simulink model "simulink"  (R2015a)
settings: Solver=ode4  StartTime=0.0  StopTime=inf  FixedStep=1e-3  RelTol=1e-3
values from neighbouring files (symbols this model uses):
  b_end1 = 0.5*(k_end1*Cyl1.m)^0.5    [m-script.m]
  b_end2 = 0.5*(k_end2*Cyl2.m)^0.5    [m-script.m]
  b_end3 = 0.5*(k_end3*Cyl3.m)^0.5    [m-script.m]
  b_end4 = 0.5*(k_end4*Cyl4.m)^0.5    [m-script.m]
  Cyl1_b = 40000    [m-script.m]
  Cyl1_Fc = 20514    [m-script.m]
  Cyl1_Fs = 22360    [m-script.m]
  Cyl1_K = 20000    [m-script.m]
  Cyl1_vs = 0.8    [m-script.m]
  Cyl2_b = 30000    [m-script.m]
  Cyl2_Fc = 14950    [m-script.m]
  Cyl2_Fs = 16125    [m-script.m]
  Cyl2_K = 20000    [m-script.m]
  Cyl2_vs = 0.8    [m-script.m]
  Cyl3_b = 30000    [m-script.m]
  Cyl3_Fc = 14996    [m-script.m]
  Cyl3_Fs = 16340    [m-script.m]
  Cyl3_K = 20000    [m-script.m]
  Cyl3_vs = 0.8    [m-script.m]
  Cyl4_b = 8500    [m-script.m]
  Cyl4_Fc = 4570    [m-script.m]
  Cyl4_Fs = 4945    [m-script.m]
  Cyl4_K = 20000    [m-script.m]
  Cyl4_vs = 0.8    [m-script.m]
  k_end1 = (pr_Ps*Cyl1.A_A)/v1    [m-script.m]
  k_end2 = (pr_Ps*Cyl2.A_A)/v2    [m-script.m]
  k_end3 = (pr_Ps*Cyl3.A_A)/v3    [m-script.m]
  k_end4 = (pr_Ps*Cyl4.A_A)/v4    [m-script.m]
  pr_Ps = 215e5    (= 21500000)    [m-script.m]
  sampleTime = 0.001    [m-script.m]
  Valve_eta = 0.989    [m-script.m]
  Valve_omega = 40.5    [m-script.m]
undefined symbols (not defined in the file or in its folder): Cyl, Cyl1, Cyl2, Cyl3, Cyl4, Cylinder2, Cylinder3, Cylinder4, Extention1, Extention2, Lift, Link1, Pillar, Pinion, Piston2, Piston3, Piston4, Rack, Tilt, Valve, X, Y, Z
undefined symbols (not defined in the file): Valve1, Valve2, Valve3, Valve4
libraries: sm_lib x72, simulink x32, nesl_utility x20, simulink_extras x3, xpcrtudplib x2, xpcobsoletelib x2
(part 1 of 4)
settings Model: CovModelRefEnable=off  Creator=Lakshmi  LastModifiedBy=IHA2700
settings SolverCC: EnableConcurrentExecution=on
settings DataIOCC: LimitDataPoints=off  SaveFormat=Dataset
settings OptimizationCC: BlockReduction=off  OptimizeBlockIOStorage=off  BufferReuse=off  GlobalBufferReuse=off  ExpressionFolding=off  LocalBlockOutputs=off
settings HardwareCC: ProdIntDivRoundTo=Zero  ProdEndianess=LittleEndian  ProdLongLongMode=on  ProdHWDeviceType=Generic->32-bit x86 compatible
settings ModelReferenceCC: PropagateSignalLabelsOutOfModel=on
settings RTWCC: SystemTargetFile=slrt.tlc  TemplateMakefile=slrt_default_tmf  Description=Simulink Real-Time  RTWCompilerOptimization=on
settings SimulinkRealTimeCC: GeneratePreprocessorConditionals=Disable all  xPCisModelTimeout=off
settings ConfigurationSet: Description=Simscape Multibody

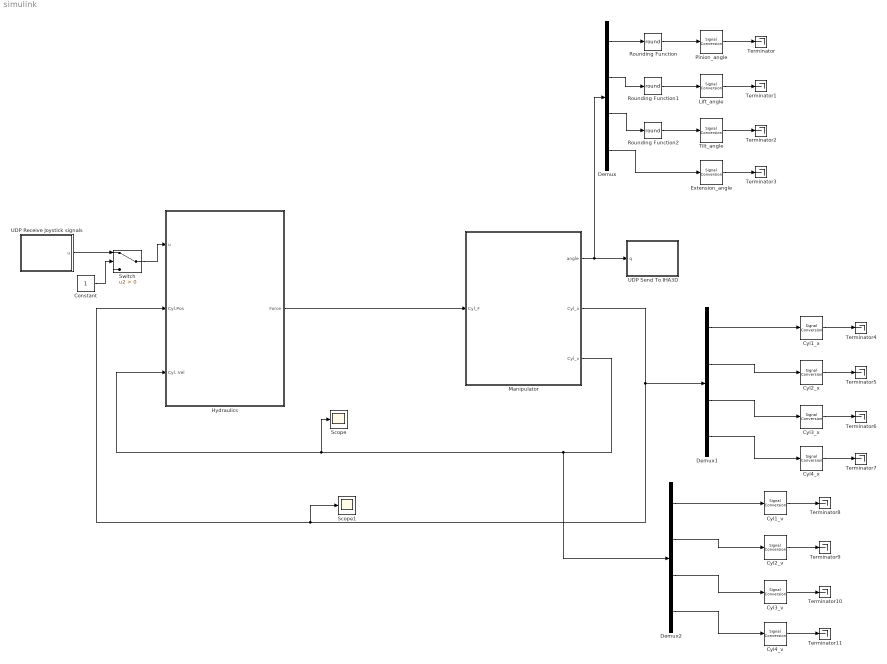
== system simulink ==
  Constant : Constant
  Cyl1_v : SignalConversion
  Cyl1_x : SignalConversion
  Cyl2_v : SignalConversion
  Cyl2_x : SignalConversion
  Cyl3_v : SignalConversion
  Cyl3_x : SignalConversion
  Cyl4_v : SignalConversion
  Cyl4_x : SignalConversion
  Demux : Demux
  Demux1 : Demux
  Demux2 : Demux
  Extension_angle : SignalConversion
  Hydraulics : Subsystem
  Lift_angle : SignalConversion
  Manipulator : Subsystem
  Pinion_angle : SignalConversion
  Rounding Function : Rounding  Operator=round
  Rounding Function1 : Rounding  Operator=round
  Rounding Function2 : Rounding  Operator=round
  Scope : Scope
      settings: YMin=-0.00025  YMax=0.00175  SaveName=ScopeData25
  Scope1 : Scope
      settings: YMin=2.77556e-17  YMax=0.7  SaveName=ScopeData26
  Switch : Switch  Criteria=u2 > Threshold
  Terminator{,1..11} (12 alike) : Terminator
  Tilt_angle : SignalConversion
  UDP Receive Joystick signals : Subsystem
  UDP Send To IHA3D : Subsystem
  wires:
  Hydraulics/1(Force) -> Manipulator/1(Cyl_F)
  Manipulator/1("angle ") -> Demux/1, UDP Send To IHA3D/1(q)
  UDP Receive Joystick signals/1(u) -> Switch/1
  Switch/1 -> Hydraulics/1(u)
  Constant/1 -> Switch/2
  Demux/1 -> Rounding Function/1
  Demux/2 -> Rounding Function1/1
  Demux/3 -> Rounding Function2/1
  Rounding Function/1 -> Pinion_angle/1
  Rounding Function1/1 -> Lift_angle/1
  Rounding Function2/1 -> Tilt_angle/1
  Demux/4 -> Extension_angle/1
  Pinion_angle/1 -> Terminator/1
  Lift_angle/1 -> Terminator1/1
  Tilt_angle/1 -> Terminator2/1
  Extension_angle/1 -> Terminator3/1
  Manipulator/2(Cyl_x) -> Demux1/1, Scope1/1, Hydraulics/2(Cyl.Pos)
  Demux1/1 -> Cyl1_x/1
  Demux1/2 -> Cyl2_x/1
  Demux1/3 -> Cyl3_x/1
  Demux1/4 -> Cyl4_x/1
  Cyl1_x/1 -> Terminator4/1
  Cyl2_x/1 -> Terminator5/1
  Cyl3_x/1 -> Terminator6/1
  Cyl4_x/1 -> Terminator7/1
  Manipulator/3(Cyl_v) -> Demux2/1, Scope/1, Hydraulics/3(Cyl. Vel)
  Demux2/1 -> Cyl1_v/1
  Demux2/2 -> Cyl2_v/1
  Demux2/3 -> Cyl3_v/1
  Demux2/4 -> Cyl4_v/1
  Cyl1_v/1 -> Terminator8/1
  Cyl2_v/1 -> Terminator9/1
  Cyl3_v/1 -> Terminator10/1
  Cyl4_v/1 -> Terminator11/1

== system simulink/Hydraulics ==
  u : Inport
  Cyl.Pos : Inport  Port=2
  Cyl. Vel : Inport  Port=3
  Constant1 : Constant  Value=pr_Ps
  Cylinder 1 : Subsystem
  Cylinder 2 : Subsystem
  Cylinder 3 : Subsystem
  Cylinder 5 : Subsystem
  Demux : Demux
  Demux1 : Demux
  Demux2 : Demux
  Mux : Mux
  Scope{,1..7} (8 alike) : Scope
      Scope settings: SaveName=ScopeData27
      Scope1 settings: YMin=0.65972  YMax=0.659805  SaveName=ScopeData28
      Scope2 settings: YMin=0.23118  YMax=0.23126  SaveName=ScopeData29
      Scope3 settings: YMin=0.359998  YMax=0.36  SaveName=ScopeData36
      Scope4 settings: SaveName=ScopeData37
      Scope5 settings: SaveName=ScopeData38
      Scope6 settings: YMin=9.845e-06  YMax=9.955e-06  SaveName=ScopeData39
      Scope7 settings: YMin=-3.8e-07  YMax=-2.5e-07  SaveName=ScopeData40
  Force : Outport
  wires:
  Cylinder 5/1(" Force") -> Mux/4
  Cyl.Pos/1 -> Demux/1
  Demux2/3 -> Scope5/1, Cylinder 3/2(v)
  Cylinder 3/1(" Force") -> Mux/3
  Cylinder 1/1(" Force") -> Mux/1
  Cylinder 2/1(" Force") -> Mux/2
  Demux/1 -> Scope3/1, Cylinder 1/3(x)
  Cyl. Vel/1 -> Demux2/1
  Demux/2 -> Scope2/1, Cylinder 2/3(x)
  Demux2/4 -> Scope4/1, Cylinder 5/2(v)
  Demux/3 -> Scope1/1, Cylinder 3/1(x)
  Mux/1 -> Force/1
  Demux2/2 -> Scope6/1, Cylinder 2/2(v)
  Demux1/1 -> Cylinder 1/1(u)
  Demux1/2 -> Cylinder 2/1(u)
  Demux1/3 -> Cylinder 3/3(u)
  Demux1/4 -> Cylinder 5/3(u)
  u/1 -> Demux1/1
  Constant1/1 -> Cylinder 2/4(Supply.Pr), Cylinder 1/4(Supply.Pr), Cylinder 5/4(Supply.Pr), Cylinder 3/4(Supply.Pr)
  Demux/4 -> Scope/1, Cylinder 5/1(x)
  Demux2/1 -> Scope7/1, Cylinder 1/2(v)

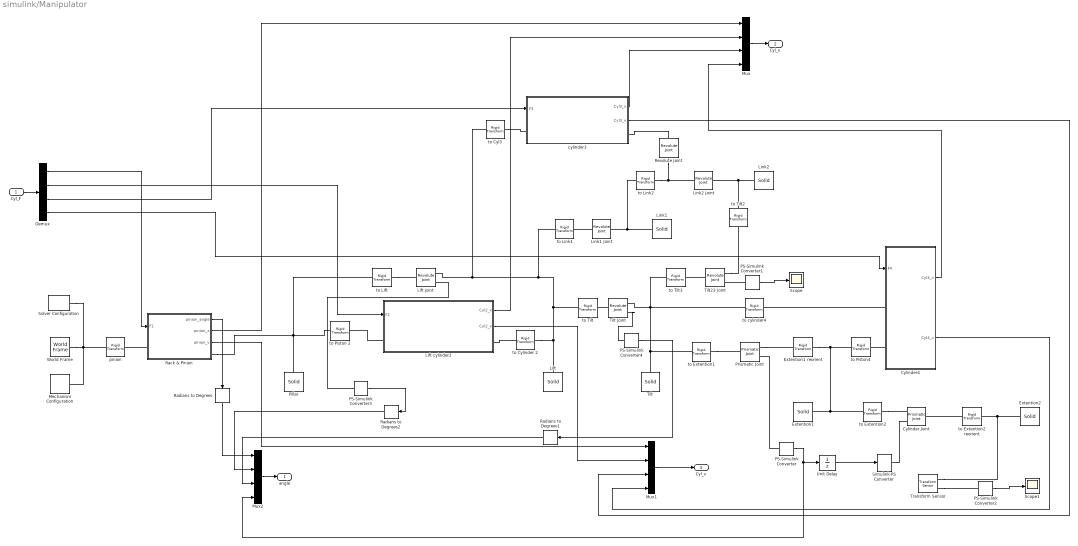
== system simulink/Manipulator ==
  Cyl_F : Inport
  Cylinder Joint : sm_lib/Joints/Prismatic Joint  SenseConstraintForce=off  SenseConstraintForceX=off  SenseConstraintForceY=off  SenseConstraintForceZ=off  SenseConstraintTorque=off  SenseConstraintTorqueX=off  SenseConstraintTorqueY=off  SenseConstraintTorqueZ=off  SenseTotalForce=off  SenseTotalForceX=off  SenseTotalForceY=off  SenseTotalForceZ=off  SenseTotalTorque=off  SenseTotalTorqueX=off  SenseTotalTorqueY=off  SenseTotalTorqueZ=off  CompositeWrenchDir=FollowerOnBase  CompositeWrenchFrame=BaseFrame  EquilibriumPosition=0  EquilibriumPositionUnits=m  SpringStiffness=0  SpringStiffnessUnits=N/m  DampingCoefficient=0  DampingCoefficientUnits=N/(m/s)  TorqueActuationMode=ComputedTorque  MotionActuationMode=InputMotion  SensePosition=off  SenseVelocity=off  SenseAcceleration=off  SenseTorqueForce=off  PositionTargetSpecify=off  PositionTargetPriority=High  PositionTargetValue=0  PositionTargetValueUnits=m  VelocityTargetSpecify=off  VelocityTargetPriority=High  VelocityTargetValue=0  VelocityTargetValueUnits=m/s  BlockFunction=simmechanics.library.joints.prismatic_joint
  Cylinder4 : Subsystem
  Demux : Demux
  Extention1 : sm_lib/Body Elements/Solid  InertiaType=Custom  Mass=Extention1.m  MassUnits=kg  CenterOfMass=Extention1.cm  CenterOfMassUnits=m  MomentsOfInertia=[1 1 1]  MomentsOfInertiaUnits=kg*m^2  ProductsOfInertia=[0 0 0]  ProductsOfInertiaUnits=kg*m^2  DensityBased=on  Density=1000  DensityUnits=kg/(m^3)  GraphicType=FromGeometry  MarkerShape=Sphere  MarkerSize=10  MarkerSizeUnits=m  GraphicVisPropType=SimpleVisualProperties  GraphicDiffuseColor=Extention1.rgb  GraphicSpecularColor=[0.5 0.5 0.5 1.0]  GraphicAmbientColor=[0.15 0.15 0.15 1.0]  GraphicEmissiveColor=[0.0 0.0 0.0 1.0]  GraphicShininess=75  GraphicOpacity=1.0  GeometryShape=GeneralExtrusion  RectangleSize=[1 1]  RectangleSizeUnits=m  BrickDimensions=[1 1 1]  BrickDimensionUnits=m  CylinderRadius=1  CylinderRadiusUnits=m  CylinderLength=1  CylinderLengthUnits=m  SphereRadius=1  SphereRadiusUnits=m  EllipsoidRadii=[1 1 1]  EllipsoidRadiiUnits=m  ExtrusionCrossSection=Extention1.c  ExtrusionCrossSectionUnits=m  ExtrusionLength=Extention1.l+0.1  ExtrusionLengthUnits=m  PolygonNumSides=3  PolygonOuterRadius=1  PolygonOuterRadiusUnits=m  ExtGeomFileType=STEP  ExtGeomFileUnits=m  RevolutionCrossSection=[1 1; 1 -1; 2 -1; 2 1]  RevolutionCrossSectionUnits=m  RevolutionExtent=Full  RevolutionAngle=180  RevolutionAngleUnits=deg  BlockFunction=simmechanics.library.body_elements.solid
  Extention1 reorient : sm_lib/Frames and Transforms/Rigid Transform  TranslationMethod=None  TranslationLengthUnit=m  TranslationStandardAxis=+Z  TranslationStandardOffset=0  TranslationCartesianOffset=Extention1.j  TranslationROffset=0  TranslationROffsetUnits=m  TranslationZOffset=0  TranslationZOffsetUnits=m  TranslationThetaOffset=0  TranslationThetaOffsetUnits=deg  RotationMethod=StandardAxis  RotationAngleUnits=deg  RotationStandardAxis=+Y  RotationAngle=-90  RotationArbitraryAxis=[0 0 1]  FollAlignAxisA=+X  BaseAlignAxisA=+Y  FollAlignAxisB=+Y  BaseAlignAxisB=+Z  RotationMatrix=[1 0 0; 0 1 0; 0 0 1]  BlockFunction=simmechanics.library.frames_transforms.rigid_transform
  Extention2 : sm_lib/Body Elements/Solid  InertiaType=Custom  Mass=Extention2.m  MassUnits=kg  CenterOfMass=Extention2.cm  CenterOfMassUnits=m  MomentsOfInertia=[1 1 1]  MomentsOfInertiaUnits=kg*m^2  ProductsOfInertia=[0 0 0]  ProductsOfInertiaUnits=kg*m^2  DensityBased=on  Density=1000  DensityUnits=kg/(m^3)  GraphicType=FromGeometry  MarkerShape=Sphere  MarkerSize=10  MarkerSizeUnits=m  GraphicVisPropType=SimpleVisualProperties  GraphicDiffuseColor=[Extention2.rgb]  GraphicSpecularColor=[0.5 0.5 0.5 1.0]  GraphicAmbientColor=[0.15 0.15 0.15 1.0]  GraphicEmissiveColor=[0.0 0.0 0.0 1.0]  GraphicShininess=75  GraphicOpacity=1.0  GeometryShape=GeneralExtrusion  RectangleSize=[1 1]  RectangleSizeUnits=m  BrickDimensions=[1 1 1]  BrickDimensionUnits=m  CylinderRadius=1  CylinderRadiusUnits=m  CylinderLength=1  CylinderLengthUnits=m  SphereRadius=1  SphereRadiusUnits=m  EllipsoidRadii=[1 1 1]  EllipsoidRadiiUnits=m  ExtrusionCrossSection=Extention2.c  ExtrusionCrossSectionUnits=m  ExtrusionLength=Extention2.l  ExtrusionLengthUnits=m  PolygonNumSides=3  PolygonOuterRadius=1  PolygonOuterRadiusUnits=m  ExtGeomFileType=STEP  ExtGeomFileUnits=m  RevolutionCrossSection=[1 1; 1 -1; 2 -1; 2 1]  RevolutionCrossSectionUnits=m  RevolutionExtent=Full  RevolutionAngle=180  RevolutionAngleUnits=deg  BlockFunction=simmechanics.library.body_elements.solid
  Lift : sm_lib/Body Elements/Solid  InertiaType=Custom  Mass=Lift.m  MassUnits=kg  CenterOfMass=[Lift.cm]  CenterOfMassUnits=m  MomentsOfInertia=[1 1 1]  MomentsOfInertiaUnits=kg*m^2  ProductsOfInertia=[0 0 0]  ProductsOfInertiaUnits=kg*m^2  DensityBased=on  Density=1000  DensityUnits=kg/(m^3)  GraphicType=FromGeometry  MarkerShape=Sphere  MarkerSize=10  MarkerSizeUnits=m  GraphicVisPropType=SimpleVisualProperties  GraphicDiffuseColor=[Lift.rgb]  GraphicSpecularColor=[0.5 0.5 0.5 1.0]  GraphicAmbientColor=[0.15 0.15 0.15 1.0]  GraphicEmissiveColor=[0.0 0.0 0.0 1.0]  GraphicShininess=75  GraphicOpacity=1.0  GeometryShape=GeneralExtrusion  RectangleSize=[1 1]  RectangleSizeUnits=m  BrickDimensions=[1 1 1]  BrickDimensionUnits=m  CylinderRadius=1  CylinderRadiusUnits=m  CylinderLength=1  CylinderLengthUnits=m  SphereRadius=1  SphereRadiusUnits=m  EllipsoidRadii=[1 1 1]  EllipsoidRadiiUnits=m  ExtrusionCrossSection=[Lift.c]  ExtrusionCrossSectionUnits=m  ExtrusionLength=Lift.l  ExtrusionLengthUnits=m  PolygonNumSides=3  PolygonOuterRadius=1  PolygonOuterRadiusUnits=m  ExtGeomFileType=STEP  ExtGeomFileUnits=m  RevolutionCrossSection=[1 1; 1 -1; 2 -1; 2 1]  RevolutionCrossSectionUnits=m  RevolutionExtent=Full  RevolutionAngle=180  RevolutionAngleUnits=deg  BlockFunction=simmechanics.library.body_elements.solid
  Lift cylinder2 : Subsystem
  Lift joint : sm_lib/Joints/Revolute Joint  SenseConstraintForce=off  SenseConstraintForceX=off  SenseConstraintForceY=off  SenseConstraintForceZ=off  SenseConstraintTorque=off  SenseConstraintTorqueX=off  SenseConstraintTorqueY=off  SenseConstraintTorqueZ=off  SenseTotalForce=off  SenseTotalForceX=off  SenseTotalForceY=off  SenseTotalForceZ=off  SenseTotalTorque=off  SenseTotalTorqueX=off  SenseTotalTorqueY=off  SenseTotalTorqueZ=off  CompositeWrenchDir=FollowerOnBase  CompositeWrenchFrame=BaseFrame  EquilibriumPosition=0  EquilibriumPositionUnits=deg  SpringStiffness=0  SpringStiffnessUnits=N*m/deg  DampingCoefficient=0  DampingCoefficientUnits=N*m/(deg/s)  TorqueActuationMode=NoTorque  MotionActuationMode=ComputedMotion  SensePosition=on  SenseVelocity=off  SenseAcceleration=off  SenseTorqueForce=off  PositionTargetSpecify=on  PositionTargetPriority=High  PositionTargetValue=0  PositionTargetValueUnits=deg  VelocityTargetSpecify=off  VelocityTargetPriority=High  VelocityTargetValue=0  VelocityTargetValueUnits=deg/s  BlockFunction=simmechanics.library.joints.revolute_joint
  Link1 : sm_lib/Body Elements/Solid  InertiaType=Custom  Mass=Link1.m  MassUnits=kg  CenterOfMass=Link1.cm  CenterOfMassUnits=m  MomentsOfInertia=[1 1 1]  MomentsOfInertiaUnits=kg*m^2  ProductsOfInertia=[0 0 0]  ProductsOfInertiaUnits=kg*m^2  DensityBased=on  Density=1000  DensityUnits=kg/(m^3)  GraphicType=FromGeometry  MarkerShape=Sphere  MarkerSize=10  MarkerSizeUnits=m  GraphicVisPropType=SimpleVisualProperties  GraphicDiffuseColor=Lift.rgb  GraphicSpecularColor=[0.5 0.5 0.5 1.0]  GraphicAmbientColor=[0.15 0.15 0.15 1.0]  GraphicEmissiveColor=[0.0 0.0 0.0 1.0]  GraphicShininess=75  GraphicOpacity=1.0  GeometryShape=GeneralExtrusion  RectangleSize=[1 1]  RectangleSizeUnits=m  BrickDimensions=[1 1 1]  BrickDimensionUnits=m  CylinderRadius=1  CylinderRadiusUnits=m  CylinderLength=1  CylinderLengthUnits=m  SphereRadius=1  SphereRadiusUnits=m  EllipsoidRadii=[1 1 1]  EllipsoidRadiiUnits=m  ExtrusionCrossSection=Link1.c  ExtrusionCrossSectionUnits=m  ExtrusionLength=Link1.l  ExtrusionLengthUnits=m  PolygonNumSides=3  PolygonOuterRadius=1  PolygonOuterRadiusUnits=m  ExtGeomFileType=STEP  ExtGeomFileUnits=m  RevolutionCrossSection=[1 1; 1 -1; 2 -1; 2 1]  RevolutionCrossSectionUnits=m  RevolutionExtent=Full  RevolutionAngle=180  RevolutionAngleUnits=deg  BlockFunction=simmechanics.library.body_elements.solid
  Link1 Joint : sm_lib/Joints/Revolute Joint  SenseConstraintForce=off  SenseConstraintForceX=off  SenseConstraintForceY=off  SenseConstraintForceZ=off  SenseConstraintTorque=off  SenseConstraintTorqueX=off  SenseConstraintTorqueY=off  SenseConstraintTorqueZ=off  SenseTotalForce=off  SenseTotalForceX=off  SenseTotalForceY=off  SenseTotalForceZ=off  SenseTotalTorque=off  SenseTotalTorqueX=off  SenseTotalTorqueY=off  SenseTotalTorqueZ=off  CompositeWrenchDir=FollowerOnBase  CompositeWrenchFrame=BaseFrame  EquilibriumPosition=0  EquilibriumPositionUnits=deg  SpringStiffness=0  SpringStiffnessUnits=N*m/deg  DampingCoefficient=0  DampingCoefficientUnits=N*m/(deg/s)  TorqueActuationMode=NoTorque  MotionActuationMode=ComputedMotion  SensePosition=off  SenseVelocity=off  SenseAcceleration=off  SenseTorqueForce=off  PositionTargetSpecify=on  PositionTargetPriority=Low  PositionTargetValue=90  PositionTargetValueUnits=deg  VelocityTargetSpecify=off  VelocityTargetPriority=High  VelocityTargetValue=0  VelocityTargetValueUnits=deg/s  BlockFunction=simmechanics.library.joints.revolute_joint
  Link2 : sm_lib/Body Elements/Solid  InertiaType=Custom  Mass=Link1.m  MassUnits=kg  CenterOfMass=Link1.cm  CenterOfMassUnits=m  MomentsOfInertia=[1 1 1]  MomentsOfInertiaUnits=kg*m^2  ProductsOfInertia=[0 0 0]  ProductsOfInertiaUnits=kg*m^2  DensityBased=on  Density=1000  DensityUnits=kg/(m^3)  GraphicType=FromGeometry  MarkerShape=Sphere  MarkerSize=10  MarkerSizeUnits=m  GraphicVisPropType=SimpleVisualProperties  GraphicDiffuseColor=Lift.rgb  GraphicSpecularColor=[0.5 0.5 0.5 1.0]  GraphicAmbientColor=[0.15 0.15 0.15 1.0]  GraphicEmissiveColor=[0.0 0.0 0.0 1.0]  GraphicShininess=75  GraphicOpacity=1.0  GeometryShape=GeneralExtrusion  RectangleSize=[1 1]  RectangleSizeUnits=m  BrickDimensions=[1 1 1]  BrickDimensionUnits=m  CylinderRadius=1  CylinderRadiusUnits=m  CylinderLength=1  CylinderLengthUnits=m  SphereRadius=1  SphereRadiusUnits=m  EllipsoidRadii=[1 1 1]  EllipsoidRadiiUnits=m  ExtrusionCrossSection=Link2.c  ExtrusionCrossSectionUnits=m  ExtrusionLength=Link2.l  ExtrusionLengthUnits=m  PolygonNumSides=3  PolygonOuterRadius=1  PolygonOuterRadiusUnits=m  ExtGeomFileType=STEP  ExtGeomFileUnits=m  RevolutionCrossSection=[1 1; 1 -1; 2 -1; 2 1]  RevolutionCrossSectionUnits=m  RevolutionExtent=Full  RevolutionAngle=180  RevolutionAngleUnits=deg  BlockFunction=simmechanics.library.body_elements.solid
  Link2 Joint : sm_lib/Joints/Revolute Joint  SenseConstraintForce=off  SenseConstraintForceX=off  SenseConstraintForceY=off  SenseConstraintForceZ=off  SenseConstraintTorque=off  SenseConstraintTorqueX=off  SenseConstraintTorqueY=off  SenseConstraintTorqueZ=off  SenseTotalForce=off  SenseTotalForceX=off  SenseTotalForceY=off  SenseTotalForceZ=off  SenseTotalTorque=off  SenseTotalTorqueX=off  SenseTotalTorqueY=off  SenseTotalTorqueZ=off  CompositeWrenchDir=FollowerOnBase  CompositeWrenchFrame=BaseFrame  EquilibriumPosition=0  EquilibriumPositionUnits=deg  SpringStiffness=0  SpringStiffnessUnits=N*m/deg  DampingCoefficient=0  DampingCoefficientUnits=N*m/(deg/s)  TorqueActuationMode=NoTorque  MotionActuationMode=ComputedMotion  SensePosition=off  SenseVelocity=off  SenseAcceleration=off  SenseTorqueForce=off  PositionTargetSpecify=on  PositionTargetPriority=Low  PositionTargetValue=0  PositionTargetValueUnits=deg  VelocityTargetSpecify=off  VelocityTargetPriority=High  VelocityTargetValue=0  VelocityTargetValueUnits=deg/s  BlockFunction=simmechanics.library.joints.revolute_joint
  Mechanism Configuration : sm_lib/Utilities/Mechanism Configuration  UniformGravity=Constant  GravityVector=[0 -9.80665 0 ]  GravityUnits=m/s^2  LinearizationDelta=0.001  BlockFunction=simmechanics.library.utilities.mechanism_configuration
  Mux : Mux
  Mux1 : Mux
  Mux2 : Mux
  PS-Simulink Converter{,1..4} (5 alike) : nesl_utility/PS-Simulink Converter  PhysicalDomain=network_engine_domain  SubClassName=ps_output  LeftPortType=input  RightPortType=output  PseudoPeriodic=off  Frequencies=[]  Unit=1  AffineConversion=off
  Pillar : sm_lib/Body Elements/Solid  InertiaType=Custom  Mass=Pillar.m  MassUnits=kg  CenterOfMass=[Pillar.cm]  CenterOfMassUnits=m  MomentsOfInertia=[1 1 1]  MomentsOfInertiaUnits=kg*m^2  ProductsOfInertia=[0 0 0]  ProductsOfInertiaUnits=kg*m^2  DensityBased=on  Density=1000  DensityUnits=kg/(m^3)  GraphicType=FromGeometry  MarkerShape=Sphere  MarkerSize=10  MarkerSizeUnits=m  GraphicVisPropType=SimpleVisualProperties  GraphicDiffuseColor=[Pillar.rgb]  GraphicSpecularColor=[0.5 0.5 0.5 1.0]  GraphicAmbientColor=[0.15 0.15 0.15 1.0]  GraphicEmissiveColor=[0.0 0.0 0.0 1.0]  GraphicShininess=75  GraphicOpacity=1.0  GeometryShape=GeneralExtrusion  RectangleSize=[1 1]  RectangleSizeUnits=m  BrickDimensions=[1 1 1]  BrickDimensionUnits=m  CylinderRadius=1  CylinderRadiusUnits=m  CylinderLength=1  CylinderLengthUnits=m  SphereRadius=1  SphereRadiusUnits=m  EllipsoidRadii=[1 1 1]  EllipsoidRadiiUnits=m  ExtrusionCrossSection=[Pillar.c]  ExtrusionCrossSectionUnits=m  ExtrusionLength=Pillar.l  ExtrusionLengthUnits=m  PolygonNumSides=3  PolygonOuterRadius=1  PolygonOuterRadiusUnits=m  ExtGeomFileType=STEP  ExtGeomFileUnits=m  RevolutionCrossSection=[1 1; 1 -1; 2 -1; 2 1]  RevolutionCrossSectionUnits=m  RevolutionExtent=Full  RevolutionAngle=180  RevolutionAngleUnits=deg  BlockFunction=simmechanics.library.body_elements.solid
  Prismatic Joint : sm_lib/Joints/Prismatic Joint  SenseConstraintForce=off  SenseConstraintForceX=off  SenseConstraintForceY=off  SenseConstraintForceZ=off  SenseConstraintTorque=off  SenseConstraintTorqueX=off  SenseConstraintTorqueY=off  SenseConstraintTorqueZ=off  SenseTotalForce=off  SenseTotalForceX=off  SenseTotalForceY=off  SenseTotalForceZ=off  SenseTotalTorque=off  SenseTotalTorqueX=off  SenseTotalTorqueY=off  SenseTotalTorqueZ=off  CompositeWrenchDir=FollowerOnBase  CompositeWrenchFrame=BaseFrame  EquilibriumPosition=0  EquilibriumPositionUnits=m  SpringStiffness=0  SpringStiffnessUnits=N/m  DampingCoefficient=0  DampingCoefficientUnits=N/(m/s)  TorqueActuationMode=NoTorque  MotionActuationMode=ComputedMotion  SensePosition=on  SenseVelocity=off  SenseAcceleration=off  SenseTorqueForce=off  PositionTargetSpecify=off  PositionTargetPriority=High  PositionTargetValue=0  PositionTargetValueUnits=m  VelocityTargetSpecify=off  VelocityTargetPriority=High  VelocityTargetValue=0  VelocityTargetValueUnits=m/s  BlockFunction=simmechanics.library.joints.prismatic_joint
  Rack & Pinion : Subsystem
  Radians to Degrees : simulink_extras/Transformations/Radians to Degrees
  Radians to Degrees1 : simulink_extras/Transformations/Radians to Degrees
  Radians to Degrees2 : simulink_extras/Transformations/Radians to Degrees
  Revolute Joint : sm_lib/Joints/Revolute Joint  SenseConstraintForce=off  SenseConstraintForceX=off  SenseConstraintForceY=off  SenseConstraintForceZ=off  SenseConstraintTorque=off  SenseConstraintTorqueX=off  SenseConstraintTorqueY=off  SenseConstraintTorqueZ=off  SenseTotalForce=off  SenseTotalForceX=off  SenseTotalForceY=off  SenseTotalForceZ=off  SenseTotalTorque=off  SenseTotalTorqueX=off  SenseTotalTorqueY=off  SenseTotalTorqueZ=off  CompositeWrenchDir=FollowerOnBase  CompositeWrenchFrame=BaseFrame  EquilibriumPosition=0  EquilibriumPositionUnits=deg  SpringStiffness=0  SpringStiffnessUnits=N*m/deg  DampingCoefficient=0  DampingCoefficientUnits=N*m/(deg/s)  TorqueActuationMode=NoTorque  MotionActuationMode=ComputedMotion  SensePosition=off  SenseVelocity=off  SenseAcceleration=off  SenseTorqueForce=off  PositionTargetSpecify=off  PositionTargetPriority=High  PositionTargetValue=0  PositionTargetValueUnits=deg  VelocityTargetSpecify=off  VelocityTargetPriority=High  VelocityTargetValue=0  VelocityTargetValueUnits=deg/s  BlockFunction=simmechanics.library.joints.revolute_joint
  Scope : Scope
      settings: YMin=1.03622  YMax=1.05162
  Scope1 : Scope
      settings: YMin=-0.52066  YMax=1.46246
  Simulink-PS Converter : nesl_utility/Simulink-PS Converter  PhysicalDomain=network_engine_domain  SubClassName=ps_input  LeftPortType=input  RightPortType=output  PseudoPeriodic=off  Frequencies=[]  NoiseDistribution=none  NoiseParameters=[]  Unit=1  AffineConversion=off  InputFiltering=off  SimscapeFilterOrder=1  InputFilterTimeConstant=0.001  UdotUserProvided=1
  Solver Configuration : nesl_utility/Solver Configuration  PhysicalDomain=network_engine_domain  SubClassName=solver  LeftPortType=input  RightPortType=generic  Accelerate=off  Tones=[]  Harmonics=[]  SimulateNoise=off  Profile=off  UseLocalSampling=off  EnableSwitchedLinearOptims=on  FrequencyDomain=off  UseCCode=off  RelTol=0.001  AbsTol=1e-06  MinStep=1e-09  ToWorkspace=off  RevertToSquareIcSolve=off  NumHomotopyIterations=100  DoDC=off  ResidualTolerance=1e-09  UseLocalSolver=off  LocalSolverChoice=NE_BACKWARD_EULER_ADVANCER  LocalSolverSampleTime=0.001  DoFixedCost=off  MaxNonlinIter=3  MaxModeIter=2  LinearAlgebra=Sparse  DelaysMemoryBudget=1024  AutomaticFiltering=on  FilteringTimeConstant=0.001
  Tilt : sm_lib/Body Elements/Solid  InertiaType=Custom  Mass=Tilt.m  MassUnits=kg  CenterOfMass=Tilt.cm  CenterOfMassUnits=m  MomentsOfInertia=[1 1 1]  MomentsOfInertiaUnits=kg*m^2  ProductsOfInertia=[0 0 0]  ProductsOfInertiaUnits=kg*m^2  DensityBased=on  Density=1000  DensityUnits=kg/(m^3)  GraphicType=FromGeometry  MarkerShape=Sphere  MarkerSize=10  MarkerSizeUnits=m  GraphicVisPropType=SimpleVisualProperties  GraphicDiffuseColor=Tilt.rgb  GraphicSpecularColor=[0.5 0.5 0.5 1.0]  GraphicAmbientColor=[0.15 0.15 0.15 1.0]  GraphicEmissiveColor=[0.0 0.0 0.0 1.0]  GraphicShininess=75  GraphicOpacity=1.0  GeometryShape=GeneralExtrusion  RectangleSize=[1 1]  RectangleSizeUnits=m  BrickDimensions=[1 1 1]  BrickDimensionUnits=m  CylinderRadius=1  CylinderRadiusUnits=m  CylinderLength=1  CylinderLengthUnits=m  SphereRadius=1  SphereRadiusUnits=m  EllipsoidRadii=[1 1 1]  EllipsoidRadiiUnits=m  ExtrusionCrossSection=Tilt.c  ExtrusionCrossSectionUnits=m  ExtrusionLength=Tilt.l  ExtrusionLengthUnits=m  PolygonNumSides=3  PolygonOuterRadius=1  PolygonOuterRadiusUnits=m  ExtGeomFileType=STEP  ExtGeomFileUnits=m  RevolutionCrossSection=[1 1; 1 -1; 2 -1; 2 1]  RevolutionCrossSectionUnits=m  RevolutionExtent=Full  RevolutionAngle=180  RevolutionAngleUnits=deg  BlockFunction=simmechanics.library.body_elements.solid
  Tilt Joint : sm_lib/Joints/Revolute Joint  SenseConstraintForce=off  SenseConstraintForceX=off  SenseConstraintForceY=off  SenseConstraintForceZ=off  SenseConstraintTorque=off  SenseConstraintTorqueX=off  SenseConstraintTorqueY=off  SenseConstraintTorqueZ=off  SenseTotalForce=off  SenseTotalForceX=off  SenseTotalForceY=off  SenseTotalForceZ=off  SenseTotalTorque=off  SenseTotalTorqueX=off  SenseTotalTorqueY=off  SenseTotalTorqueZ=off  CompositeWrenchDir=FollowerOnBase  CompositeWrenchFrame=BaseFrame  EquilibriumPosition=0  EquilibriumPositionUnits=deg  SpringStiffness=0  SpringStiffnessUnits=N*m/deg  DampingCoefficient=0  DampingCoefficientUnits=N*m/(deg/s)  TorqueActuationMode=NoTorque  MotionActuationMode=ComputedMotion  SensePosition=on  SenseVelocity=off  SenseAcceleration=off  SenseTorqueForce=off  PositionTargetSpecify=off  PositionTargetPriority=Low  PositionTargetValue=90  PositionTargetValueUnits=deg  VelocityTargetSpecify=off  VelocityTargetPriority=High  VelocityTargetValue=0  VelocityTargetValueUnits=deg/s  BlockFunction=simmechanics.library.joints.revolute_joint
  Tilt23 Joint : sm_lib/Joints/Revolute Joint  SenseConstraintForce=off  SenseConstraintForceX=off  SenseConstraintForceY=off  SenseConstraintForceZ=off  SenseConstraintTorque=off  SenseConstraintTorqueX=off  SenseConstraintTorqueY=off  SenseConstraintTorqueZ=off  SenseTotalForce=off  SenseTotalForceX=off  SenseTotalForceY=off  SenseTotalForceZ=off  SenseTotalTorque=off  SenseTotalTorqueX=off  SenseTotalTorqueY=off  SenseTotalTorqueZ=off  CompositeWrenchDir=FollowerOnBase  CompositeWrenchFrame=BaseFrame  EquilibriumPosition=0  EquilibriumPositionUnits=deg  SpringStiffness=0  SpringStiffnessUnits=N*m/deg  DampingCoefficient=0  DampingCoefficientUnits=N*m/(deg/s)  TorqueActuationMode=NoTorque  MotionActuationMode=ComputedMotion  SensePosition=on  SenseVelocity=off  SenseAcceleration=off  SenseTorqueForce=off  PositionTargetSpecify=off  PositionTargetPriority=High  PositionTargetValue=0  PositionTargetValueUnits=deg  VelocityTargetSpecify=off  VelocityTargetPriority=High  VelocityTargetValue=0  VelocityTargetValueUnits=deg/s  BlockFunction=simmechanics.library.joints.revolute_joint
  Transform Sensor : sm_lib/Frames and Transforms/Transform Sensor  MeasurementFrame=World  SenseAngle=off  SenseAxis=off  SenseAngle1=off  SenseAngle2=off  SenseAngle3=off  SenseQ=off  SenseR=off  SenseOmegaX=off  SenseOmegaY=off  SenseOmegaZ=off  SenseOmega1=off  SenseOmega2=off  SenseOmega3=off  SenseQDot=off  SenseRDot=off  SenseAlphaX=off  SenseAlphaY=off  SenseAlphaZ=off  SenseAlpha1=off  SenseAlpha2=off  SenseAlpha3=off  SenseQDDot=off  SenseRDDot=off  SenseX=off  SenseY=off  SenseZ=off  SenseRad=off  SenseAzim=off  SenseDist=off  SenseInc=off  SenseXDot=off  SenseYDot=off  SenseZDot=off  SenseRadDot=off  SenseAzimDot=off  SenseDistDot=on  SenseIncDot=off  SenseXDDot=off  SenseYDDot=off  SenseZDDot=off  SenseRadDDot=off  SenseAzimDDot=off  SenseDistDDot=off  SenseIncDDot=off  BlockFunction=simmechanics.library.frames_transforms.transform_sensor
  Unit Delay : UnitDelay  SampleTime=-1
  World Frame : sm_lib/Frames and Transforms/World Frame  BlockFunction=simmechanics.library.frames_transforms.world_frame
  cylinder3 : Subsystem
  pinion : sm_lib/Frames and Transforms/Rigid Transform  TranslationMethod=Cartesian  TranslationLengthUnit=m  TranslationStandardAxis=+Z  TranslationStandardOffset=0  TranslationCartesianOffset=Pinion.j/2  TranslationROffset=0  TranslationROffsetUnits=m  TranslationZOffset=0  TranslationZOffsetUnits=m  TranslationThetaOffset=0  TranslationThetaOffsetUnits=deg  RotationMethod=None  RotationAngleUnits=deg  RotationStandardAxis=+Z  RotationAngle=0.0  RotationArbitraryAxis=[0 0 1]  FollAlignAxisA=+X  BaseAlignAxisA=+Y  FollAlignAxisB=+Y  BaseAlignAxisB=+Z  RotationMatrix=[1 0 0; 0 1 0; 0 0 1]  BlockFunction=simmechanics.library.frames_transforms.rigid_transform
  to Cyl3 : sm_lib/Frames and Transforms/Rigid Transform  TranslationMethod=Cartesian  TranslationLengthUnit=m  TranslationStandardAxis=+Z  TranslationStandardOffset=0  TranslationCartesianOffset=Cylinder3.j  TranslationROffset=0  TranslationROffsetUnits=m  TranslationZOffset=0  TranslationZOffsetUnits=m  TranslationThetaOffset=0  TranslationThetaOffsetUnits=deg  RotationMethod=None  RotationAngleUnits=deg  RotationStandardAxis=+Z  RotationAngle=0.0  RotationArbitraryAxis=[0 0 1]  FollAlignAxisA=+X  BaseAlignAxisA=+Y  FollAlignAxisB=+Y  BaseAlignAxisB=+Z  RotationMatrix=[1 0 0; 0 1 0; 0 0 1]  BlockFunction=simmechanics.library.frames_transforms.rigid_transform
  to Cylinder 2 : sm_lib/Frames and Transforms/Rigid Transform  TranslationMethod=Cartesian  TranslationLengthUnit=m  TranslationStandardAxis=+Z  TranslationStandardOffset=0  TranslationCartesianOffset=[Cylinder2.pos]  TranslationROffset=0  TranslationROffsetUnits=m  TranslationZOffset=0  TranslationZOffsetUnits=m  TranslationThetaOffset=0  TranslationThetaOffsetUnits=deg  RotationMethod=None  RotationAngleUnits=deg  RotationStandardAxis=+Z  RotationAngle=0.0  RotationArbitraryAxis=[0 0 1]  FollAlignAxisA=+X  BaseAlignAxisA=+Y  FollAlignAxisB=+Y  BaseAlignAxisB=+Z  RotationMatrix=[1 0 0; 0 1 0; 0 0 1]  BlockFunction=simmechanics.library.frames_transforms.rigid_transform
  to Extention1 : sm_lib/Frames and Transforms/Rigid Transform  TranslationMethod=Cartesian  TranslationLengthUnit=m  TranslationStandardAxis=+Z  TranslationStandardOffset=0  TranslationCartesianOffset=Extention1.j  TranslationROffset=0  TranslationROffsetUnits=m  TranslationZOffset=0  TranslationZOffsetUnits=m  TranslationThetaOffset=0  TranslationThetaOffsetUnits=deg  RotationMethod=StandardAxis  RotationAngleUnits=deg  RotationStandardAxis=+Y  RotationAngle=90  RotationArbitraryAxis=[0 0 1]  FollAlignAxisA=+X  BaseAlignAxisA=+Y  FollAlignAxisB=+Y  BaseAlignAxisB=+Z  RotationMatrix=[1 0 0; 0 1 0; 0 0 1]  BlockFunction=simmechanics.library.frames_transforms.rigid_transform
  to Extention2 : sm_lib/Frames and Transforms/Rigid Transform  TranslationMethod=Cartesian  TranslationLengthUnit=m  TranslationStandardAxis=+Z  TranslationStandardOffset=0  TranslationCartesianOffset=Extention2.j  TranslationROffset=0  TranslationROffsetUnits=m  TranslationZOffset=0  TranslationZOffsetUnits=m  TranslationThetaOffset=0  TranslationThetaOffsetUnits=deg  RotationMethod=StandardAxis  RotationAngleUnits=deg  RotationStandardAxis=+Y  RotationAngle=90  RotationArbitraryAxis=[0 0 1]  FollAlignAxisA=+X  BaseAlignAxisA=+Y  FollAlignAxisB=+Y  BaseAlignAxisB=+Z  RotationMatrix=[1 0 0; 0 1 0; 0 0 1]  BlockFunction=simmechanics.library.frames_transforms.rigid_transform
  to Extention2 reorient : sm_lib/Frames and Transforms/Rigid Transform  TranslationMethod=None  TranslationLengthUnit=m  TranslationStandardAxis=+Z  TranslationStandardOffset=0  TranslationCartesianOffset=Extention1.j  TranslationROffset=0  TranslationROffsetUnits=m  TranslationZOffset=0  TranslationZOffsetUnits=m  TranslationThetaOffset=0  TranslationThetaOffsetUnits=deg  RotationMethod=StandardAxis  RotationAngleUnits=deg  RotationStandardAxis=+Y  RotationAngle=-90  RotationArbitraryAxis=[0 0 1]  FollAlignAxisA=+X  BaseAlignAxisA=+Y  FollAlignAxisB=+Y  BaseAlignAxisB=+Z  RotationMatrix=[1 0 0; 0 1 0; 0 0 1]  BlockFunction=simmechanics.library.frames_transforms.rigid_transform
  to Lift : sm_lib/Frames and Transforms/Rigid Transform  TranslationMethod=Cartesian  TranslationLengthUnit=m  TranslationStandardAxis=+Z  TranslationStandardOffset=0  TranslationCartesianOffset=[Lift.j]  TranslationROffset=0  TranslationROffsetUnits=m  TranslationZOffset=0  TranslationZOffsetUnits=m  TranslationThetaOffset=0  TranslationThetaOffsetUnits=deg  RotationMethod=None  RotationAngleUnits=deg  RotationStandardAxis=+Z  RotationAngle=0.0  RotationArbitraryAxis=[0 0 1]  FollAlignAxisA=+X  BaseAlignAxisA=+Y  FollAlignAxisB=+Y  BaseAlignAxisB=+Z  RotationMatrix=[1 0 0; 0 1 0; 0 0 1]  BlockFunction=simmechanics.library.frames_transforms.rigid_transform
  to Link1 : sm_lib/Frames and Transforms/Rigid Transform  TranslationMethod=Cartesian  TranslationLengthUnit=m  TranslationStandardAxis=+Z  TranslationStandardOffset=0  TranslationCartesianOffset=Link1.j  TranslationROffset=0  TranslationROffsetUnits=m  TranslationZOffset=0  TranslationZOffsetUnits=m  TranslationThetaOffset=0  TranslationThetaOffsetUnits=deg  RotationMethod=None  RotationAngleUnits=deg  RotationStandardAxis=+Z  RotationAngle=0.0  RotationArbitraryAxis=[0 0 1]  FollAlignAxisA=+X  BaseAlignAxisA=+Y  FollAlignAxisB=+Y  BaseAlignAxisB=+Z  RotationMatrix=[1 0 0; 0 1 0; 0 0 1]  BlockFunction=simmechanics.library.frames_transforms.rigid_transform
  to Link2 : sm_lib/Frames and Transforms/Rigid Transform  TranslationMethod=Cartesian  TranslationLengthUnit=m  TranslationStandardAxis=+Z  TranslationStandardOffset=0  TranslationCartesianOffset=Link2.j  TranslationROffset=0  TranslationROffsetUnits=m  TranslationZOffset=0  TranslationZOffsetUnits=m  TranslationThetaOffset=0  TranslationThetaOffsetUnits=deg  RotationMethod=None  RotationAngleUnits=deg  RotationStandardAxis=+Z  RotationAngle=0.0  RotationArbitraryAxis=[0 0 1]  FollAlignAxisA=+X  BaseAlignAxisA=+Y  FollAlignAxisB=+Y  BaseAlignAxisB=+Z  RotationMatrix=[1 0 0; 0 1 0; 0 0 1]  BlockFunction=simmechanics.library.frames_transforms.rigid_transform
  to Piston 2 : sm_lib/Frames and Transforms/Rigid Transform  TranslationMethod=Cartesian  TranslationLengthUnit=m  TranslationStandardAxis=+Z  TranslationStandardOffset=0  TranslationCartesianOffset=[Piston2.pos]  TranslationROffset=0  TranslationROffsetUnits=m  TranslationZOffset=0  TranslationZOffsetUnits=m  TranslationThetaOffset=0  TranslationThetaOffsetUnits=deg  RotationMethod=None  RotationAngleUnits=deg  RotationStandardAxis=+Z  RotationAngle=0.0  RotationArbitraryAxis=[0 0 1]  FollAlignAxisA=+X  BaseAlignAxisA=+Y  FollAlignAxisB=+Y  BaseAlignAxisB=+Z  RotationMatrix=[1 0 0; 0 1 0; 0 0 1]  BlockFunction=simmechanics.library.frames_transforms.rigid_transform
  to Piston4 : sm_lib/Frames and Transforms/Rigid Transform  TranslationMethod=Cartesian  TranslationLengthUnit=m  TranslationStandardAxis=+Z  TranslationStandardOffset=0  TranslationCartesianOffset=Piston4.pos  TranslationROffset=0  TranslationROffsetUnits=m  TranslationZOffset=0  TranslationZOffsetUnits=m  TranslationThetaOffset=0  TranslationThetaOffsetUnits=deg  RotationMethod=None  RotationAngleUnits=deg  RotationStandardAxis=+Z  RotationAngle=0.0  RotationArbitraryAxis=[0 0 1]  FollAlignAxisA=+X  BaseAlignAxisA=+Y  FollAlignAxisB=+Y  BaseAlignAxisB=+Z  RotationMatrix=[1 0 0; 0 1 0; 0 0 1]  BlockFunction=simmechanics.library.frames_transforms.rigid_transform
  to Tilt : sm_lib/Frames and Transforms/Rigid Transform  TranslationMethod=Cartesian  TranslationLengthUnit=m  TranslationStandardAxis=+Z  TranslationStandardOffset=0  TranslationCartesianOffset=Tilt.j  TranslationROffset=0  TranslationROffsetUnits=m  TranslationZOffset=0  TranslationZOffsetUnits=m  TranslationThetaOffset=0  TranslationThetaOffsetUnits=deg  RotationMethod=None  RotationAngleUnits=deg  RotationStandardAxis=+Z  RotationAngle=0.0  RotationArbitraryAxis=[0 0 1]  FollAlignAxisA=+X  BaseAlignAxisA=+Y  FollAlignAxisB=+Y  BaseAlignAxisB=+Z  RotationMatrix=[1 0 0; 0 1 0; 0 0 1]  BlockFunction=simmechanics.library.frames_transforms.rigid_transform
  to Tilt2 : sm_lib/Frames and Transforms/Rigid Transform  TranslationMethod=Cartesian  TranslationLengthUnit=m  TranslationStandardAxis=+Z  TranslationStandardOffset=0  TranslationCartesianOffset=Tilt2.j  TranslationROffset=0  TranslationROffsetUnits=m  TranslationZOffset=0  TranslationZOffsetUnits=m  TranslationThetaOffset=0  TranslationThetaOffsetUnits=deg  RotationMethod=None  RotationAngleUnits=deg  RotationStandardAxis=+Z  RotationAngle=0.0  RotationArbitraryAxis=[0 0 1]  FollAlignAxisA=+X  BaseAlignAxisA=+Y  FollAlignAxisB=+Y  BaseAlignAxisB=+Z  RotationMatrix=[1 0 0; 0 1 0; 0 0 1]  BlockFunction=simmechanics.library.frames_transforms.rigid_transform
  to Tilt3 : sm_lib/Frames and Transforms/Rigid Transform  TranslationMethod=Cartesian  TranslationLengthUnit=m  TranslationStandardAxis=+Z  TranslationStandardOffset=0  TranslationCartesianOffset=Tilt3.j  TranslationROffset=0  TranslationROffsetUnits=m  TranslationZOffset=0  TranslationZOffsetUnits=m  TranslationThetaOffset=0  TranslationThetaOffsetUnits=deg  RotationMethod=None  RotationAngleUnits=deg  RotationStandardAxis=+Z  RotationAngle=0.0  RotationArbitraryAxis=[0 0 1]  FollAlignAxisA=+X  BaseAlignAxisA=+Y  FollAlignAxisB=+Y  BaseAlignAxisB=+Z  RotationMatrix=[1 0 0; 0 1 0; 0 0 1]  BlockFunction=simmechanics.library.frames_transforms.rigid_transform
  to cylinder4 : sm_lib/Frames and Transforms/Rigid Transform  TranslationMethod=Cartesian  TranslationLengthUnit=m  TranslationStandardAxis=+Z  TranslationStandardOffset=0  TranslationCartesianOffset=Cylinder4.pos  TranslationROffset=0  TranslationROffsetUnits=m  TranslationZOffset=0  TranslationZOffsetUnits=m  TranslationThetaOffset=0  TranslationThetaOffsetUnits=deg  RotationMethod=None  RotationAngleUnits=deg  RotationStandardAxis=+Z  RotationAngle=0.0  RotationArbitraryAxis=[0 0 1]  FollAlignAxisA=+X  BaseAlignAxisA=+Y  FollAlignAxisB=+Y  BaseAlignAxisB=+Z  RotationMatrix=[1 0 0; 0 1 0; 0 0 1]  BlockFunction=simmechanics.library.frames_transforms.rigid_transform
  "angle " : Outport
  Cyl_x : Outport  Port=2
  Cyl_v : Outport  Port=3
  wires:
  Demux/3 -> cylinder3/1(F3)
  Demux/1 -> Rack & Pinion/1(F1)
  Demux/2 -> Lift cylinder2/1(F2)
  Demux/4 -> Cylinder4/1(F4)
  Cyl_F/1 -> Demux/1
  Rack & Pinion/2(pinion_x) -> Mux/1
  cylinder3/1(Cyl3_x) -> Mux/3
  Lift cylinder2/1(Cyl2_x) -> Mux/2
  Cylinder4/1(Cyl4_x) -> Mux/4
  Rack & Pinion/1(pinion_angle) -> Radians to Degrees/1
  Rack & Pinion/3(pinion_v) -> Mux1/1
  Lift cylinder2/2(Cyl2_v) -> Mux1/2
  Cylinder4/2(Cyl4_v) -> Mux1/4
  cylinder3/2(Cyl3_v) -> Mux1/3
  Mux1/1 -> Cyl_v/1
  Mux/1 -> Cyl_x/1
  PS-Simulink Converter1/1 -> Scope/1
  PS-Simulink Converter2/1 -> Scope1/1
  Mux2/1 -> "angle "/1
  PS-Simulink Converter3/1 -> Radians to Degrees2/1
  PS-Simulink Converter4/1 -> Radians to Degrees1/1
  PS-Simulink Converter/1 -> Mux2/4, Unit Delay/1
  Radians to Degrees2/1 -> Mux2/2
  Radians to Degrees/1 -> Mux2/1
  Radians to Degrees1/1 -> Mux2/3
  Unit Delay/1 -> Simulink-PS Converter/1
  connections:
  to Cylinder 2/LConn1 -- to Link1/LConn1 -- to Cyl3/LConn1 -- Lift joint/RConn1 -- to Tilt/LConn1 -- Lift/RConn1
  to Lift/RConn1 -- Lift joint/LConn1
  Lift cylinder2/RConn1 -- to Cylinder 2/RConn1
  Link1 Joint/LConn1 -- to Link1/RConn1
  Lift cylinder2/LConn1 -- to Piston 2/RConn1
  Link1/RConn1 -- to Link2/LConn1 -- Link1 Joint/RConn1
  to Link2/RConn1 -- Link2 Joint/LConn1 -- Revolute Joint/LConn1
  Tilt Joint/LConn1 -- to Tilt/RConn1
  Prismatic Joint/RConn1 -- Extention1 reorient/LConn1
  to Extention2 reorient/LConn1 -- Cylinder Joint/RConn1
  cylinder3/RConn1 -- Revolute Joint/RConn1
  to Extention1/RConn1 -- Prismatic Joint/LConn1
  Extention2/RConn1 -- Transform Sensor/RConn1 -- to Extention2 reorient/RConn1
  Solver Configuration/RConn1 -- pinion/LConn1 -- Mechanism Configuration/RConn1 -- World Frame/RConn1
  to Extention2/RConn1 -- Cylinder Joint/LConn1
  Extention1 reorient/RConn1 -- to Extention2/LConn1 -- Extention1/RConn1 -- to Piston4/LConn1
  Tilt23 Joint/RConn1 -- to Tilt2/RConn1
  Link2/RConn1 -- Link2 Joint/RConn1 -- to Tilt2/LConn1
  Tilt23 Joint/LConn1 -- to Tilt3/RConn1
  cylinder3/LConn1 -- to Cyl3/RConn1
  Tilt/RConn1 -- to Extention1/LConn1 -- to Tilt3/LConn1 -- Tilt Joint/RConn1 -- to cylinder4/LConn1
  Cylinder4/LConn2 -- to Piston4/RConn1
  Cylinder4/LConn1 -- to cylinder4/RConn1
  Pillar/RConn1 -- to Piston 2/LConn1 -- to Lift/LConn1 -- Rack & Pinion/RConn1
  PS-Simulink Converter/LConn1 -- Prismatic Joint/RConn2
  Rack & Pinion/LConn1 -- pinion/RConn1
  PS-Simulink Converter1/LConn1 -- Tilt23 Joint/RConn2
  Transform Sensor/RConn2 -- PS-Simulink Converter2/LConn1
  PS-Simulink Converter3/LConn1 -- Lift joint/RConn2
  Tilt Joint/RConn2 -- PS-Simulink Converter4/LConn1
  Simulink-PS Converter/RConn1 -- Cylinder Joint/LConn2

== system simulink/UDP Receive Joystick signals ==
  Mux : Mux
  Receive signals from Joytick : xpcrtudplib/Legacy UDP/Receive   ipAddress=192.168.10.1  ipPort=55550  width=32  vblLen=off  sampletime=sampleTime
  Terminator : Terminator
  Unpack : xpcobsoletelib/Utilities/Unpack   dimensions={[1],[1],[1],[1]}  datatypes={'double','double','double','double'}  byteAlign=1
  u : Outport
  wires:
  Mux/1 -> u/1
  Unpack/4 -> Mux/4
  Unpack/3 -> Mux/3
  Unpack/2 -> Mux/2
  Unpack/1 -> Mux/1
  Receive signals from Joytick/1 -> Unpack/1
  Receive signals from Joytick/2 -> Terminator/1

== system simulink/UDP Send To IHA3D ==
  note: Frequency rate:
      | How often UDP message is sent
      | 1: every sample time
      | 2: every second sample time
      | 3: every third sample time
      | 4: etc....
  q : Inport
  Enabled Subsystem : Subsystem  TreatAsAtomicUnit=on
  Frequency rate : Constant  Value=5
  Subsystem : Subsystem
  wires:
  q/1 -> Enabled Subsystem/1(q)
  Frequency rate/1 -> Subsystem/1(freq)
  Subsystem/1(enable) -> Enabled Subsystem/Enable

== system simulink/Hydraulics/Cylinder 1 ==
  u : Inport
  v : Inport  Port=2
  x : Inport  Port=3
  Supply.Pr : Inport  Port=4
  4/3 Valve : Subsystem
  Constant : Constant  Value=0
  Cylinder : Subsystem
  Terminator : Terminator
  Terminator1 : Terminator
  " Force" : Outport
  wires:
  v/1 -> Cylinder/4(dx/dt)
  Cylinder/3(F) -> " Force"/1
  4/3 Valve/4(Q_B) -> Cylinder/2(Q_B)
  Constant/1 -> 4/3 Valve/3(p_T)
  4/3 Valve/3(Q_A) -> Cylinder/1(Q_A)
  4/3 Valve/2(Q_T) -> Terminator1/1
  Supply.Pr/1 -> 4/3 Valve/2(p_S)
  4/3 Valve/1(Q_P) -> Terminator/1
  x/1 -> Cylinder/3(x)
  u/1 -> 4/3 Valve/4(u)
  Cylinder/1(p_A) -> 4/3 Valve/1(p_A)
  Cylinder/2(p_B) -> 4/3 Valve/5(p_B)

== system simulink/Hydraulics/Cylinder 2 ==
  note: s
  u : Inport
  v : Inport  Port=2
  x : Inport  Port=3
  Supply.Pr : Inport  Port=4
  4/3 Valve : Subsystem
  Constant : Constant  Value=0
  Cylinder : Subsystem
  Terminator : Terminator
  Terminator1 : Terminator
  " Force" : Outport
  wires:
  v/1 -> Cylinder/4(dx/dt)
  Cylinder/3(F) -> " Force"/1
  Constant/1 -> 4/3 Valve/3(p_T)
  4/3 Valve/2(Q_T) -> Terminator1/1
  Supply.Pr/1 -> 4/3 Valve/2(p_S)
  4/3 Valve/1(Q_P) -> Terminator/1
  x/1 -> Cylinder/3(x)
  u/1 -> 4/3 Valve/4(u)
  4/3 Valve/3(Q_A) -> Cylinder/1(Q_A)
  4/3 Valve/4(Q_B) -> Cylinder/2(Q_B)
  Cylinder/1(p_A) -> 4/3 Valve/1(p_A)
  Cylinder/2(p_B) -> 4/3 Valve/5(p_B)

== system simulink/Hydraulics/Cylinder 3 ==
  x : Inport
  v : Inport  Port=2
  u : Inport  Port=3
  Supply.Pr : Inport  Port=4
  4/3 Valve : Subsystem
  Constant : Constant  Value=0
  Cylinder : Subsystem
  Terminator : Terminator
  Terminator1 : Terminator
  " Force" : Outport
  wires:
  v/1 -> Cylinder/4(dx/dt)
  Cylinder/3(F) -> " Force"/1
  Constant/1 -> 4/3 Valve/3(p_T)
  4/3 Valve/2(Q_T) -> Terminator1/1
  Supply.Pr/1 -> 4/3 Valve/2(p_S)
  4/3 Valve/1(Q_P) -> Terminator/1
  x/1 -> Cylinder/3(x)
  u/1 -> 4/3 Valve/4(u)
  4/3 Valve/3(Q_A) -> Cylinder/1(Q_A)
  4/3 Valve/4(Q_B) -> Cylinder/2(Q_B)
  Cylinder/2(p_B) -> 4/3 Valve/5(p_B)
  Cylinder/1(p_A) -> 4/3 Valve/1(p_A)

== system simulink/Hydraulics/Cylinder 5 ==
  x : Inport
  v : Inport  Port=2
  u : Inport  Port=3
  Supply.Pr : Inport  Port=4
  4/3 Valve : Subsystem
  Constant : Constant  Value=0
  Cylinder : Subsystem
  Scope : Scope
      settings: YMin=-0.00761  YMax=0.00675  SaveName=ScopeData5
  Scope1 : Scope
      settings: YMin=-0.00461  YMax=0.00297  SaveName=ScopeData6
  Terminator : Terminator
  Terminator1 : Terminator
  " Force" : Outport
  wires:
  u/1 -> 4/3 Valve/4(u)
  x/1 -> Cylinder/3(x)
  4/3 Valve/1(Q_P) -> Terminator/1
  Supply.Pr/1 -> 4/3 Valve/2(p_S)
  4/3 Valve/2(Q_T) -> Terminator1/1
  Constant/1 -> 4/3 Valve/3(p_T)
  Cylinder/3(F) -> " Force"/1
  v/1 -> Cylinder/4(dx/dt)
  4/3 Valve/4(Q_B) -> Cylinder/2(Q_B), Scope1/1
  4/3 Valve/3(Q_A) -> Cylinder/1(Q_A), Scope/1
  Cylinder/1(p_A) -> 4/3 Valve/1(p_A)
  Cylinder/2(p_B) -> 4/3 Valve/5(p_B)
